simulink model "LKS"  (R2020a)
settings: Solver=FixedStepAuto  StartTime=0.0  StopTime=inf  RelTol=1e-3  EnableMultiTasking=on
undefined symbols (not defined in the file): gray
libraries: embdlinuxlib x2, raspberrypiBasiclib x2, dspmtrx3 x1, visionanalysis x1, simulink x1, visiongeotforms x1, visiontextngfix x1
settings Model: SimulationMode=external  Creator=Administrator  LastModifiedBy=zhengliang
settings SolverCC: PositivePriorityOrder=on  AutoInsertRateTranBlk=on
settings DataIOCC: ReturnWorkspaceOutputs=off
settings OptimizationCC: EnhancedBackFolding=on  PassReuseOutputArgsAs=Individual arguments  MaxStackSize=64  OptimizeBlockOrder=speed  DifferentSizesBufferReuse=on  OptimizationCustomize=off  EfficientTunableParamExpr=on
settings DebuggingCC: ParameterTunabilityLossMsg=error  ArithmeticOperatorsInVariantConditions=warning
settings HardwareCC: ProdBitPerPointer=32  ProdBitPerSizeT=32  ProdBitPerPtrDiffT=32  ProdLargestAtomicInteger=Long  ProdLargestAtomicFloat=Double  ProdWordSize=32  ProdHWDeviceType=ARM Compatible->ARM Cortex
settings SFSimCC: MATLABDynamicMemAlloc=off  CustomCodeUndefinedFunction=UseInterfaceOnly
settings RTWCC: SystemTargetFile=ert.tlc  HardwareBoard=Raspberry Pi  TemplateMakefile=ert_default_tmf  GenerateReport=on  Toolchain=GNU GCC Raspberry Pi  BuildConfiguration=Faster Runs  IncludeHyperlinkInReport=on  LaunchReport=on  GenerateTraceInfo=on  GenerateTraceReport=on  GenerateTraceReportSl=on  GenerateTraceReportSf=on  GenerateTraceReportEml=on
settings CodeAppCC: ForceParamTrailComments=on  IgnoreCustomStorageClasses=off  OperatorAnnotations=on  SimulinkDataObjDesc=on  SFDataObjDesc=on  InsertBlockDesc=on
settings ERTTargetCC: SupportContinuousTime=on  SupportVariableSizeSignals=on

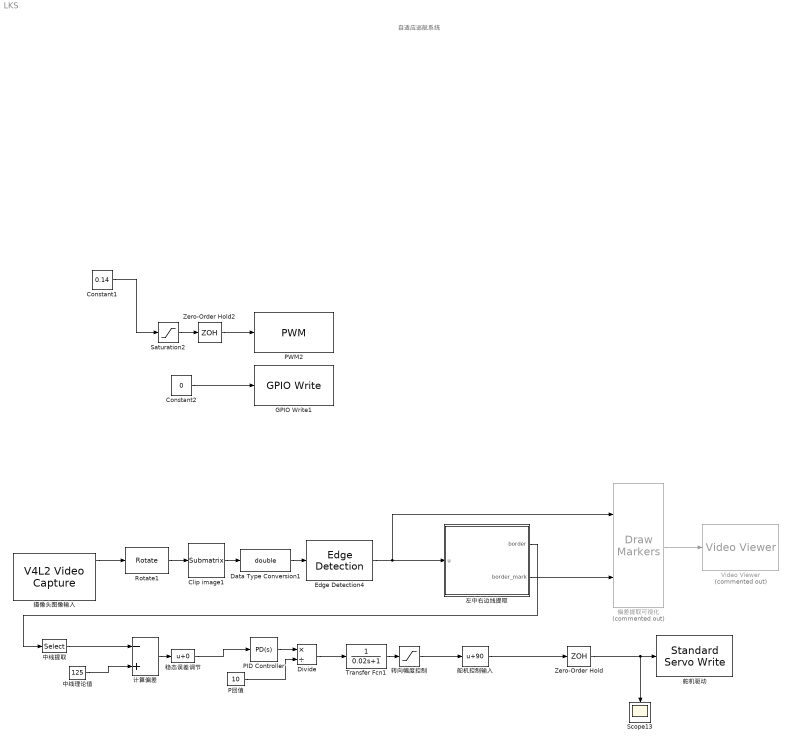
== system LKS ==
  note: 自适应巡航系统
  Clip image1 : dspmtrx3/Submatrix  RowSpan=Range of rows  RowStartMode=Index  RowStartIndex=110  RowEndMode=Index  RowEndIndex=210  ColSpan=Range of columns  ColStartMode=Index  ColStartIndex=50  ColEndMode=Index  ColEndIndex=280
  Constant1 : Constant  Value=0.14
  Constant2 : Constant  Value=0
  Data Type Conversion1 : DataTypeConversion  OutDataTypeStr=double
  Divide : Product  Inputs=*/
  Edge Detection4 : visionanalysis/Edge Detection  method=Sobel  outputType=Binary image  userDefinedThreshold=on  thresholdSource=Specify via dialog  threshold=22  thresholdTuning=1  edgeThinning=on  threshold_canny=[0.25 0.60]  autoPercent=90  sigma=1  roundingMode=Floor  overflowMode=off  prodOutputMode=Binary point scaling  prodOutputWordLength=32  prodOutputFracLength=8
      settings: SourceProductBaseCode=VP
  GPIO Write1 : embdlinuxlib/GPIO Write  board=Pi 3 Model B+  gpio=17  direction=Output  blockPlatform=Raspberry Pi
      settings: SourceProductBaseCode=SC_BEAGLEBONE_BLUE,RASPPI
  PID Controller : simulink/Continuous/PID Controller  Controller=PD  Form=Parallel  TimeDomain=Continuous-time  UseExternalTs=off  SampleTime=-1  IntegratorMethod=Forward Euler  FilterMethod=Forward Euler  ControllerParametersSource=internal  P=15  I=0.001  D=0.8  UseFilter=on  N=3  TunerSelectOption=Transfer Function Based (PID Tuner App)  InitialConditionSource=internal  InitialConditionForIntegrator=0  InitialConditionForFilter=0  DifferentiatorICPrevScaledInput=0  ExternalReset=none  TrackingMode=off  Kt=1  LimitOutput=off  UpperSaturationLimit=inf  LowerSaturationLimit=-inf  LinearizeAsGain=on  AntiWindupMode=none  Kb=1  POutMin=[]  POutMax=[]  IOutMin=[]  IOutMax=[]  DOutMin=[]  DOutMax=[]  NOutMin=[]  NOutMax=[]  SumOutMin=[]  SumOutMax=[]  SaturationOutMin=[]  SaturationOutMax=[]  PParamMin=[]  PParamMax=[]  IParamMin=[]  IParamMax=[]  DParamMin=[]  DParamMax=[]  NParamMin=[]  NParamMax=[]  KbParamMin=[]  KbParamMax=[]  KtParamMin=[]  KtParamMax=[]  KbOutMin=[]  KbOutMax=[]  KtOutMin=[]  KtOutMax=[]  IntegratorOutMin=[]  IntegratorOutMax=[]  FilterOutMin=[]  FilterOutMax=[]  SumI1OutMin=[]  SumI1OutMax=[]  SumI2OutMin=[]  SumI2OutMax=[]  SumI3OutMin=[]  SumI3OutMax=[]  SumI4OutMin=[]  SumI4OutMax=[]  SumDOutMin=[]  SumDOutMax=[]  DifferentiatorOutMin=[]  DifferentiatorOutMax=[]  FilterDiffOutCoefMin=[]  FilterDiffOutCoefMax=[]  ReciprocalOutMin=[]  ReciprocalOutMax=[]  SumDenOutMin=[]  SumDenOutMax=[]  SumNumOutMin=[]  SumNumOutMax=[]  DivideOutMin=[]  DivideOutMax=[]  UdiffTsProdOutMin=[]  UdiffTsProdOutMax=[]  NTsProdOutMin=[]  NTsProdOutMax=[]  UintegralTsProdOutMin=[]  UintegralTsProdOutMax=[]  UngainTsProdOutMin=[]  UngainTsProdOutMax=[]  IntegratorContinuousStateAttributes=''  IntegratorStateMustResolveToSignalObject=off  IntegratorRTWStateStorageClass=Auto  FilterContinuousStateAttributes=''  FilterStateMustResolveToSignalObject=off  FilterRTWStateStorageClass=Auto  ParallelPVariant=InternalParameters  IdealPVariant=Disabled  IVariant=Disabled  DVariant=InternalParameters  IntegratorVariant=Disabled  SatVariant=Disabled  AWVariant=Disabled  PCopyVariant=Disabled  TRVariant=Disabled  FdbkBlocksVariant=Forward  IdealPFdbkVariant=Disabled  SatFdbkVariant=Disabled  DerivativeFilterVariant=ContFilter  NVariant=InternalParameters  NCopyVariant=Disabled  FilterICVariant=InternalICsFilter  IntegratorICVariant=Disabled  ExternalResetVariant=Disabled  TRSumVariant=Passthrough  SumFdbkVariant=Disabled  SumVariant=Sum_PD  TsampFilterVariant=InternalTs  TsampNgainVariant=Passthrough  TsampIntegralVariant=Disabled_SignalSpec
  PWM2 : raspberrypiBasiclib/PWM  board=Pi 3 Model B  Pin_=27  Frequency=8000  blockPlatform=Raspberry Pi
      settings: SourceProductBaseCode=RASPPI
  P回值 : Constant  Value=10
  Rotate1 : visiongeotforms/Rotate  outSizeR=Expanded to fit rotated input image  src_angle=Specify via dialog  unit_angle=Degrees  angle=-pi/2  maxAngle=pi  dispImage=Top-left corner  method=Table lookup  fillVal=0  interpMethod=Bilinear  roundingMode=Nearest  overflowMode=on  prodOutputMode=Binary point scaling  prodOutputWordLength=32  prodOutputFracLength=10
      settings: LockScale=on
  Saturation2 : Saturate  UpperLimit=0.2  LowerLimit=0
  Scope13 : Scope
  Transfer Fcn1 : TransferFcn  Denominator=[0.02 1]
  Video Viewer : VideoViewer  Commented=on  colormapValue=gray(256)  FigPos=[1 862 868.8 408]
  Zero-Order Hold : ZeroOrderHold  SampleTime=0.1
  Zero-Order Hold2 : ZeroOrderHold  SampleTime=0.05
  中线提取 : Selector  NumberOfDimensions=2  InputPortWidth=3  IndexOptions=Index vector (dialog),Index vector (dialog)  Indices=[2],2  OutputSizes=1,1
  中线理论值 : Constant  Value=125
  偏差提取可视化 : visiontextngfix/Draw Markers  Commented=on  shape=Circle  size=3  fill=off  fillClrSource=Specify via dialog  display=White  intensity=200  color=[200 255 100]  opacity=0.6  viewport=Entire image  antialiasing=off  inType=Obsolete  imagePorts=One multidimensional signal  roundingMode=Floor  overflowMode=off  memoryMode=Specify word length  memoryWordLength=16  memoryFracLength=15  prodOutputMode=Binary point scaling  prodOutputWordLength=32  prodOutputFracLength=14
      settings: SourceProductBaseCode=VP
  左中右边线提取 : MATLAB Function  TreatAsAtomicUnit=on
  摄像头图像输入 : embdlinuxlib/V4L2 Video Capture  m_devName='/dev/video0'  roi=[0, 0, 640, 480]  imSizeSelection=320x240  imSize=[640, 480]  pixelFormat=RGB  pixelOrder=Planar  sampleTime=1/30  simOutput=Colorbars  blockPlatform=Raspberry Pi
      settings: SourceProductBaseCode=SC_BEAGLEBONE_BLUE,RASPPI
  稳态误差调节 : Bias
  舵机控制输入 : Bias  Bias=90
  舵机驱动 : raspberrypiBasiclib/Standard Servo Write  board=Pi 3 Model B+  Pin_=21  MinPulseDuration=0.96e-3  MaxPulseDuration=1.96e-3  blockPlatform=Raspberry Pi
      settings: SourceProductBaseCode=RASPPI
  计算偏差 : Sum  Inputs=-+
  转向幅度控制 : Saturate  UpperLimit=85  LowerLimit=-85
  wires:
  P回值/1 -> Divide/2
  Transfer Fcn1/1 -> 转向幅度控制/1
  Divide/1 -> Transfer Fcn1/1
  左中右边线提取/1(border) -> 中线提取/1
  Zero-Order Hold/1 -> 舵机驱动/1, Scope13/1
  舵机控制输入/1 -> Zero-Order Hold/1
  中线理论值/1 -> 计算偏差/2
  左中右边线提取/2(border_mark) -> 偏差提取可视化/2
  Clip image1/1 -> Data Type Conversion1/1
  Rotate1/1 -> Clip image1/1
  转向幅度控制/1 -> 舵机控制输入/1
  偏差提取可视化/1 -> Video Viewer/1
  稳态误差调节/1 -> PID Controller/1
  PID Controller/1 -> Divide/1
  Data Type Conversion1/1 -> Edge Detection4/1
  中线提取/1 -> 计算偏差/1
  摄像头图像输入/1 -> Rotate1/1
  计算偏差/1 -> 稳态误差调节/1
  Edge Detection4/1 -> 偏差提取可视化/1, 左中右边线提取/1(u)
  Constant2/1 -> GPIO Write1/1
  Saturation2/1 -> Zero-Order Hold2/1
  Zero-Order Hold2/1 -> PWM2/1
  Constant1/1 -> Saturation2/1

== matlab function LKS/左中右边线提取 ==
  data: u input; border output; border_mark output
function [border,border_mark]= fcn(u)
scan_line=[100 75 50 25];
scan_lines=length(scan_line);
border=zeros(scan_lines,3);
[~,x_max]=size(u);
x_max_2 = x_max/2;
for i=1:scan_lines
    border(i,3)= x_max;
    border(i,2)= x_max_2;
end
mid = x_max_2;
%start to scan the border
for y=1:scan_lines
    for x_left=1:mid
        if u(scan_line(y),mid-x_left+1)==1
           border(y,1)=x_max_2-x_left;
           break
        end
    end
    for x_right=1:(x_max-mid)
        if u(scan_line(y),mid+x_right-1)==1
           border(y,3)=x_max_2+x_right;
           break
        end
    end
    border(y,2)=(border(y,1)+border(y,3))/2;
    mid = border(y,2);
end
%output the border in video
border_mark =int16(zeros(scan_lines*3,2));
for y=1:scan_lines*3
    border_mark(y,2)=scan_line(fix(y/3.1+1));
    border_mark(y,1)=border(fix(y/3.1+1),rem(y+2,3)+1);
end
